simulink model "crazyflie_sim"  (R2024a)
settings: Solver=ode4  StartTime=0.0  StopTime=20.0  FixedStep=1/600  RelTol=1e-3
values from neighbouring files (symbols this model uses):
  ui_height = 1.5    [setupSim.m]
  ui_shape_id = 1    [setupSim.m]
  ui_speed = 1.0    (= 1)    [setupSim.m]
  ui_time = 20.0    (= 20)    [setupSim.m]
  ui_width = 2.0    (= 2)    [setupSim.m]
libraries: sharedutil x1
settings Model: Creator=gunna  LastModifiedBy=gunna

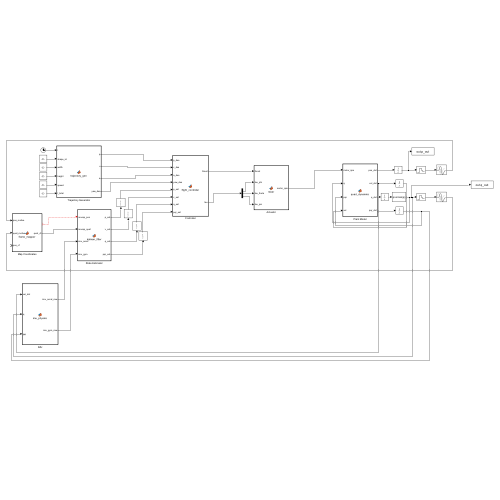
[thumbnail: Simulink's stored preview of the top-level diagram]
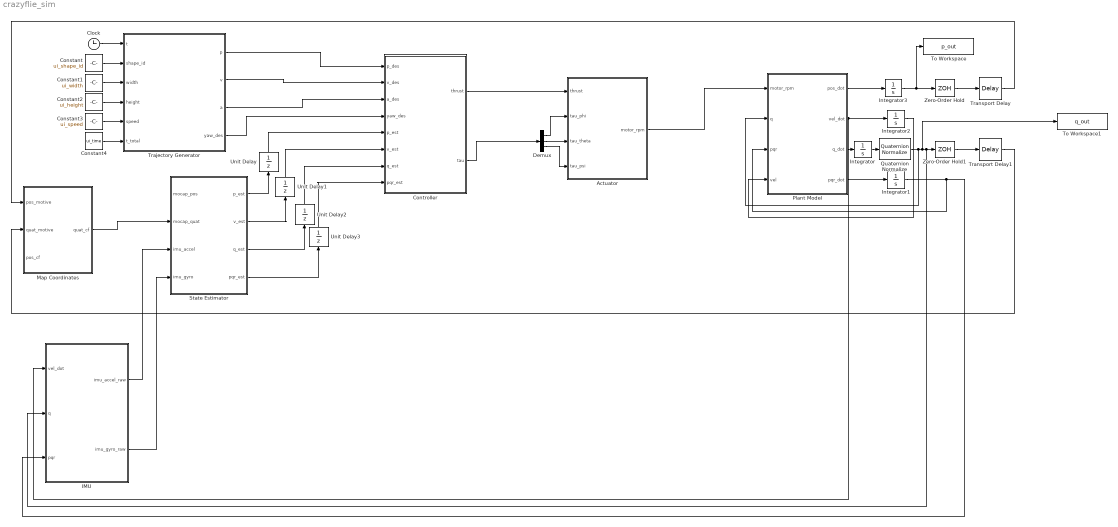
== system crazyflie_sim ==
  Actuator : MATLAB Function  TreatAsAtomicUnit=on
  Clock : Clock
  Constant : Constant  Value=ui_shape_id
  Constant1 : Constant  Value=ui_width
  Constant2 : Constant  Value=ui_height
  Constant3 : Constant  Value=ui_speed
  Constant4 : Constant  Value=ui_time
  Controller : MATLAB Function  TreatAsAtomicUnit=on
  Demux : Demux  Outputs=3
  IMU : MATLAB Function  TreatAsAtomicUnit=on
  Integrator : Integrator  InitialCondition=[1; 0; 0; 0]
  Integrator1 : Integrator  InitialCondition=[0; 0; 0]
  Integrator2 : Integrator  InitialCondition=[0; 0; 0]
  Integrator3 : Integrator  InitialCondition=[0; 0; 0]
  Map Coordinates : MATLAB Function  TreatAsAtomicUnit=on
  Plant Model : MATLAB Function  TreatAsAtomicUnit=on
  Quaternion Normalize : sharedutil/Quaternion Normalize  aMode=aMode
  State Estimator : MATLAB Function  TreatAsAtomicUnit=on
  To Workspace : ToWorkspace  VariableName=p_out  SaveFormat=Timeseries  SampleTime=-1
  To Workspace1 : ToWorkspace  VariableName=q_out  SaveFormat=Timeseries  SampleTime=-1
  Trajectory Generator : MATLAB Function  TreatAsAtomicUnit=on
  Transport Delay : TransportDelay  DelayTime=0.15
  Transport Delay1 : TransportDelay  DelayTime=0.15
  Unit Delay : UnitDelay  SampleTime=-1  HasFrameUpgradeWarning=on
  Unit Delay1 : UnitDelay  SampleTime=-1  HasFrameUpgradeWarning=on
  Unit Delay2 : UnitDelay  InitialCondition=[1; 0; 0; 0]  SampleTime=-1  HasFrameUpgradeWarning=on
  Unit Delay3 : UnitDelay  SampleTime=-1  HasFrameUpgradeWarning=on
  Zero-Order Hold : ZeroOrderHold  SampleTime=1/120
  Zero-Order Hold1 : ZeroOrderHold  SampleTime=1/120
  wires:
  Clock/1 -> Trajectory Generator/1(t)
  Constant/1 -> Trajectory Generator/2(shape_id)
  Constant1/1 -> Trajectory Generator/3(width)
  Constant2/1 -> Trajectory Generator/4(height)
  Constant3/1 -> Trajectory Generator/5(speed)
  Constant4/1 -> Trajectory Generator/6(t_total)
  Trajectory Generator/1(p) -> Controller/1(p_des)
  Trajectory Generator/2(v) -> Controller/2(v_des)
  Trajectory Generator/3(a) -> Controller/3(a_des)
  Controller/1(thrust) -> Actuator/1(thrust)
  Controller/2(tau) -> Demux/1
  Demux/1 -> Actuator/2(tau_phi)
  Demux/2 -> Actuator/3(tau_theta)
  Demux/3 -> Actuator/4(tau_psi)
  Actuator/1(motor_rpm) -> Plant Model/1(motor_rpm)
  State Estimator/1(p_est) -> Unit Delay/1
  State Estimator/2(v_est) -> Unit Delay1/1
  State Estimator/3(q_est) -> Unit Delay2/1
  State Estimator/4(pqr_est) -> Unit Delay3/1
  Plant Model/3(q_dot) -> Integrator/1
  Plant Model/2(vel_dot) -> Integrator2/1, IMU/1(vel_dot)
  Plant Model/4(pqr_dot) -> Integrator1/1
  Integrator1/1 -> Plant Model/3(pqr), IMU/3(pqr)
  Integrator2/1 -> Plant Model/4(vel)
  Quaternion Normalize/1 -> To Workspace1/1, IMU/2(q), Zero-Order Hold1/1, Plant Model/2(q)
  ? -> State Estimator/1(mocap_pos)
  Map Coordinates/1(quat_cf) -> State Estimator/2(mocap_quat)
  Plant Model/1(pos_dot) -> Integrator3/1
  Integrator3/1 -> To Workspace/1, Zero-Order Hold/1
  Zero-Order Hold/1 -> Transport Delay/1
  Transport Delay/1 -> Map Coordinates/1(pos_motive)
  Zero-Order Hold1/1 -> Transport Delay1/1
  Transport Delay1/1 -> Map Coordinates/2(quat_motive)
  IMU/2(imu_gyro_raw) -> State Estimator/4(imu_gyro)
  IMU/1(imu_accel_raw) -> State Estimator/3(imu_accel)
  Trajectory Generator/4(yaw_des) -> Controller/4(yaw_des)
  Unit Delay/1 -> Controller/5(p_est)
  Unit Delay1/1 -> Controller/6(v_est)
  Unit Delay2/1 -> Controller/7(q_est)
  Unit Delay3/1 -> Controller/8(pqr_est)
  Integrator/1 -> Quaternion Normalize/1

== matlab function crazyflie_sim/Controller ==
  data: p_des input; thrust output size=1; v_des input; a_des input; yaw_des input; p_est input; v_est input; q_est input size=4; pqr_est input size=3; tau output size=[3 1]
function [thrust, tau] = flight_controller(p_des, v_des, a_des, yaw_des, p_est, v_est, q_est, pqr_est)
    m = 0.027; g = 9.81;
    
    Kp_pos = [5.0; 5.0; 10.0]; Kd_pos = [3.0; 3.0; 5.0];
    Kp_att = [100.0; 100.0; 100.0]; Kd_att = [10.0; 10.0; 10.0];
    
    % --- OUTER LOOP: Position ---
    e_p = p_des - p_est;
    e_v = v_des - v_est;
    a_cmd = a_des + (Kp_pos .* e_p) + (Kd_pos .* e_v);
    F_des = m * (a_cmd + [0; 0; g]);
    thrust = F_des(3); 
    
    % Generate Desired Euler Angles from acceleration command
    phi_des   =  (F_des(2) / m) / g;
    theta_des = -(F_des(1) / m) / g;
    
    % Convert Desired Euler to Desired Quaternion (Z-Y-X sequence)
    % q = [cos(a/2); sin(a/2)*axis]
    cy = cos(yaw_des * 0.5); sy = sin(yaw_des * 0.5);
    cp = cos(theta_des * 0.5); sp = sin(theta_des * 0.5);
    cr = cos(phi_des * 0.5); sr = sin(phi_des * 0.5);
    
    q_des = [cr*cp*cy + sr*sp*sy;
             sr*cp*cy - cr*sp*sy;
             cr*sp*cy + sr*cp*sy;
             cr*cp*sy - sr*sp*cy];
             
    % --- INNER LOOP: Quaternion Attitude Control ---
    % Calculate Quaternion Error: q_err = q_est_conjugate * q_des
    q_est_w = q_est(1); q_est_x = -q_est(2); q_est_y = -q_est(3); q_est_z = -q_est(4); % Conjugate
    
    q_err_w = q_est_w*q_des(1) - q_est_x*q_des(2) - q_est_y*q_des(3) - q_est_z*q_des(4);
    q_err_x = q_est_w*q_des(2) + q_est_x*q_des(1) + q_est_y*q_des(4) - q_est_z*q_des(3);
    q_err_y = q_est_w*q_des(3) - q_est_x*q_des(4) + q_est_y*q_des(1) + q_est_z*q_des(2);
    q_err_z = q_est_w*q_des(4) + q_est_x*q_des(3) - q_est_y*q_des(2) + q_est_z*q_des(1);
    
    % Proportional control using the vector part of the quaternion error
    % The sign(q_err_w) ensures we always take the shortest rotational path
    e_att = sign(q_err_w) * [q_err_x; q_err_y; q_err_z];
    pqr_des = Kp_att .* e_att;
    
    % Derivative control (Rates)
    e_pqr = pqr_des - pqr_est;
    tau = Kd_att .* e_pqr; 
end

== matlab function crazyflie_sim/Trajectory Generator ==
  data: t input; p output; shape_id input; width input; height input; speed input; t_total input; v output; a output; yaw_des output
function [p, v, a, yaw_des] = trajectory_gen(t, shape_id, width, height, speed, t_total)
    % Initialize outputs to zeros
    p = zeros(3,1);
    v = zeros(3,1);
    a = zeros(3,1);
    yaw_des = 0; % Default yaw angle (radians)
    
    % Ensure time doesn't exceed total time (hold final position)
    if t > t_total
        t = t_total;
    end
    
    switch shape_id
        case 1 % HELIX (Sinusoidal 3D)
            radius = width / 2;
            omega = speed; % rad/s
            v_z = height / t_total; % Climb rate
            
            p = [radius * cos(omega * t);
                 radius * sin(omega * t);
                 v_z * t];
                 
            v = [-radius * omega * sin(omega * t);
                  radius * omega * cos(omega * t);
                  v_z];
                 
            a = [-radius * omega^2 * cos(omega * t);
                 -radius * omega^2 * sin(omega * t);
                 0];
                 
            % THE PIROUETTE: Spin exactly in sync with the helix orbit
            yaw_des = omega * t; 
                 
        case 2 % FIGURE-8 / Lissajous (Sinusoidal 2D)
            A = width / 2; % Amplitude
            wx = speed; 
            wy = 2 * speed; 
            
            p = [A * sin(wx * t);
                 A * sin(wy * t);
                 height]; 
                 
            v = [A * wx * cos(wx * t);
                 A * wy * cos(wy * t);
                 0];
                 
            a = [-A * wx^2 * sin(wx * t);
                 -A * wy^2 * sin(wy * t);
                 0];
                 
            % TANGENT POINTING: Point nose in the direction of the velocity vector
            yaw_des = atan2(v(2), v(1));
                 
        case 3 % SQUARE (Non-Sinusoidal Piecewise)
            leg_time = t_total / 4;
            v_xy = width / leg_time; 
            p(3) = height; 
            
            if t <= leg_time
                % Leg 1: Move +X
                p(1) = v_xy * t; p(2) = 0; v(1) = v_xy;
            elseif t <= 2*leg_time
                % Leg 2: Move +Y
                t_leg = t - leg_time;
                p(1) = width; p(2) = v_xy * t_leg; v(2) = v_xy;
            elseif t <= 3*leg_time
                % Leg 3: Move -X
                t_leg = t - 2*leg_time;
                p(1) = width - (v_xy * t_leg); p(2) = width; v(1) = -v_xy;
            else
                % Leg 4: Move -Y
                t_leg = t - 3*leg_time;
                p(1) = 0; p(2) = width - (v_xy * t_leg); v(2) = -v_xy;
            end
            
            % TANGENT POINTING: Snap the nose to the new leg direction
            if norm(v) > 0
                yaw_des = atan2(v(2), v(1));
            end
    end
end

== matlab function crazyflie_sim/State Estimator ==
  settings: updateMethod=DISCRETE
  data: mocap_pos input; p_est output size=[3 1]; mocap_quat input; imu_accel input; imu_gyro input; v_est output size=[3 1]; q_est output size=[4 1]; pqr_est output size=[3 1]
function [p_est, v_est, q_est, pqr_est] = kalman_filter(mocap_pos, mocap_quat, imu_accel, imu_gyro)
    persistent x_hat P
    dt = 0.01; % 100Hz loop rate
    g = 9.81;
    
    if isempty(x_hat)
        % State: [px, py, pz, vx, vy, vz, qw, qx, qy, qz]'
        x_hat = [mocap_pos; 0; 0; 0; mocap_quat]; 
        P = eye(10); 
    end
    
    % Extract current quaternion
    qw = x_hat(7); qx = x_hat(8); qy = x_hat(9); qz = x_hat(10);
    
    % Body-to-Inertial Rotation Matrix from Quaternion
    R = [1 - 2*(qy^2 + qz^2),   2*(qx*qy - qw*qz),   2*(qx*qz + qw*qy);
         2*(qx*qy + qw*qz),     1 - 2*(qx^2 + qz^2), 2*(qy*qz - qw*qx);
         2*(qx*qz - qw*qy),     2*(qy*qz + qw*qx),   1 - 2*(qx^2 + qy^2)];
         
    % Predict Velocity and Position
    accel_inertial = R * imu_accel - [0; 0; g];
    x_pred = zeros(10,1);
    x_pred(1:3) = x_hat(1:3) + x_hat(4:6) * dt;
    x_pred(4:6) = x_hat(4:6) + accel_inertial * dt;
    
    % Predict Quaternion (Quaternion Kinematics)
    p = imu_gyro(1); q_rate = imu_gyro(2); r = imu_gyro(3);
    Omega = [ 0, -p, -q_rate, -r;
              p,  0,  r, -q_rate;
             q_rate, -r,  0,  p;
              r,  q_rate, -p,  0];
              
    q_dot = 0.5 * Omega * [qw; qx; qy; qz];
    q_pred = [qw; qx; qy; qz] + q_dot * dt;
    q_pred = q_pred / norm(q_pred); % Must normalize to remain a valid rotation
    x_pred(7:10) = q_pred;
    
    % Covariance and Update steps (Simplified for brevity, assuming highly accurate Mocap)
    % In a full EKF, you would compute the 10x10 Jacobians here.
    % Since Motive is so accurate, we can use a direct complementary filter/direct injection 
    % for the update step when a packet arrives to save computational load:
    
    alpha = 0.8; % Trust factor for Mocap
    x_pred(1:3) = (1-alpha)*x_pred(1:3) + alpha*mocap_pos;
    
    % Spherical Linear Interpolation (SLERP) for Quaternions would go here, 
    % but simple injection is fine for Simulink validation:
    x_pred(7:10) = mocap_quat; 
    
    x_hat = x_pred;
    
    p_est = x_hat(1:3);
    v_est = x_hat(4:6);
    q_est = x_hat(7:10);
    pqr_est = imu_gyro; 
end

== matlab function crazyflie_sim/Actuator ==
  data: thrust input; motor_rpm output; tau_phi input; tau_theta input; tau_psi input
function motor_rpm = mixer(thrust, tau_phi, tau_theta, tau_psi)
    % Motor Layout: 1(Front-Right), 2(Back-Right), 3(Back-Left), 4(Front-Left)
    d = 0.046; % Crazyflie arm length in meters
    c_T = 3.16e-10; % Thrust coefficient (approx)
    c_Q = 5.96e-12; % Torque coefficient (approx)
    
    % Mixer matrix mapping squared RPMs (w^2) to Forces/Torques
    % [Thrust; tau_phi; tau_theta; tau_psi] = M * [w1^2; w2^2; w3^2; w4^2]
    M = [c_T,             c_T,            c_T,             c_T;
         -c_T*d/sqrt(2), -c_T*d/sqrt(2),  c_T*d/sqrt(2),   c_T*d/sqrt(2);
         -c_T*d/sqrt(2),  c_T*d/sqrt(2),  c_T*d/sqrt(2),  -c_T*d/sqrt(2);
         -c_Q,            c_Q,           -c_Q,             c_Q];
         
    % Solve for squared motor speeds
    w_squared = M \ [thrust; tau_phi; tau_theta; tau_psi];
    
    % Prevent imaginary numbers from negative commands
    w_squared = max(w_squared, 0); 
    motor_rpm = sqrt(w_squared);
end

== matlab function crazyflie_sim/Plant Model ==
  data: motor_rpm input; pos_dot output; q input; pqr input; vel input; vel_dot output; q_dot output; pqr_dot output
function [pos_dot, vel_dot, q_dot, pqr_dot] = quad_dynamics(motor_rpm, q, pqr, vel)
    % Parameters for Crazyflie 2.0
    m = 0.027; % kg
    g = 9.81; 
    J = diag([1.66e-5, 1.66e-5, 2.93e-5]); % Inertia matrix kg*m^2
    c_T = 3.16e-10; 
    
    % Reconstruct total thrust from actual RPMs
    thrust = sum(c_T * motor_rpm.^2);
    
    % Ensure the input quaternion remains normalized (prevents numerical drift)
    q = q / norm(q);
    qw = q(1); qx = q(2); qy = q(3); qz = q(4);
    
    % --- 1. Translational Kinematics ---
    pos_dot = vel;
    
    % --- 2. Translational Dynamics ---
    % Rotation matrix (Body to Inertial) derived directly from Quaternion
    R = [1 - 2*(qy^2 + qz^2),   2*(qx*qy - qw*qz),   2*(qx*qz + qw*qy);
         2*(qx*qy + qw*qz),     1 - 2*(qx^2 + qz^2), 2*(qy*qz - qw*qx);
         2*(qx*qz - qw*qy),     2*(qy*qz + qw*qx),   1 - 2*(qx^2 + qy^2)];
    
    % Newton's Second Law
    F_body = [0; 0; thrust];
    F_inertial = R * F_body - [0; 0; m*g];
    vel_dot = F_inertial / m;
    
    % --- 3. Rotational Kinematics (Quaternion Derivative) ---
    p_rate = pqr(1); q_rate = pqr(2); r_rate = pqr(3);
    
    % Skew-symmetric matrix for quaternion integration
    Omega = [      0, -p_rate, -q_rate, -r_rate;
              p_rate,       0,  r_rate, -q_rate;
              q_rate, -r_rate,       0,  p_rate;
              r_rate,  q_rate, -p_rate,       0];
              
    q_dot = 0.5 * Omega * [qw; qx; qy; qz];
    
    % --- 4. Rotational Dynamics (Euler's Equations) ---
    % Reconstruct torques from RPMs (reverse of mixer)
    d = 0.046; c_Q = 5.96e-12;
    tau_phi   = c_T * d / sqrt(2) * (-motor_rpm(1)^2 - motor_rpm(2)^2 + motor_rpm(3)^2 + motor_rpm(4)^2);
    tau_theta = c_T * d / sqrt(2) * (-motor_rpm(1)^2 + motor_rpm(2)^2 + motor_rpm(3)^2 - motor_rpm(4)^2);
    tau_psi   = c_Q * (-motor_rpm(1)^2 + motor_rpm(2)^2 - motor_rpm(3)^2 + motor_rpm(4)^2);
    tau = [tau_phi; tau_theta; tau_psi];
    
    pqr_dot = J \ (tau - cross(pqr, J * pqr));
end

== matlab function crazyflie_sim/Map Coordinates ==
  data: pos_motive input; quat_motive input; quat_cf output; pos_cf input size=3
function quat_cf  = frame_mapper(pos_motive, quat_motive, pos_cf)
    % Map Motive (Z-up, Y-forward) to Crazyflie (Z-up, X-forward)
    pos_cf = [pos_motive(2); -pos_motive(1); pos_motive(3)];
    
    % Map Quaternions (qw, qx, qy, qz)
    quat_cf = [quat_motive(1); quat_motive(3); -quat_motive(2); quat_motive(4)];
end

== matlab function crazyflie_sim/IMU ==
  data: vel_dot input; imu_accel_raw output size=[3 1]; q input; pqr input; imu_gyro_raw output size=[3 1]
function [imu_accel_raw, imu_gyro_raw] = imu_physics(vel_dot, q, pqr)
    % vel_dot: Linear acceleration from Plant (Inertial Frame)
    % q: Current Quaternion from Plant Integrator
    % pqr: Current Body Angular Rates from Plant Integrator
    
    g = 9.81;
    
    % 1. ACCELEROMETER MATH
    % Accelerometers measure "specific force" (kinematic acceleration + gravity)
    specific_force_inertial = vel_dot + [0; 0; g];
    
    % Rotate that force from the room (Inertial) to the drone (Body) frame
    qw = q(1); qx = q(2); qy = q(3); qz = q(4);
    R_trans = [1 - 2*(qy^2 + qz^2),   2*(qx*qy + qw*qz),   2*(qx*qz - qw*qy);
               2*(qx*qy - qw*qz),     1 - 2*(qx^2 + qz^2), 2*(qy*qz + qw*qx);
               2*(qx*qz + qw*qy),     2*(qy*qz - qw*qx),   1 - 2*(qx^2 + qy^2)];
               
    imu_accel_raw = R_trans * specific_force_inertial;
    
    % 2. GYROSCOPE MATH
    % The gyroscope simply senses the body rates (pqr) directly
    imu_gyro_raw = pqr;
end
